simulink model "CDMA_AWGN"  (Simulink 7.6)
settings: Solver=ode45  StartTime=0.0  StopTime=inf  RelTol=1e-3
libraries: commdigbbndpm3 x11, commseqgen2 x8, dspsigops x6, commfilt2 x6, commchan3 x2, commrandsrc2 x2, commsink2 x1
settings Model: Creator=Administrator  LastModifiedBy=Administrator

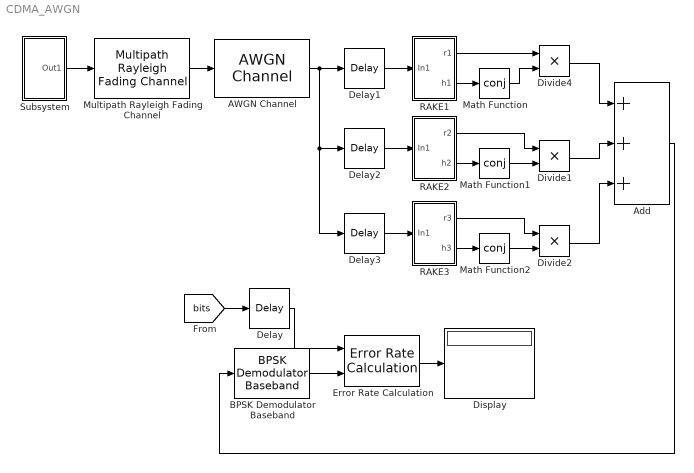
== system CDMA_AWGN ==
  AWGN Channel : commchan3/AWGN Channel  SystemSampleTime=-1  InputProcessing=Columns as channels (frame based)  seed=67  noiseMode="Signal to noise ratio  (Eb/No)"  EbNodB=4  EsNodB=10  SNRdB=10  bitsPerSym=1  Ps=1  Tsym=1e-6  variance=1
  Add : Sum  Inputs=+++
  BPSK Demodulator Baseband : commdigbbndpm3/BPSK Demodulator Baseband  DialogController=commDDGCreate  DialogControllerArgs=DataTag1  Ph=0  DecType=Hard decision  VarSource=Dialog  Variance=1  outDtype=Inherit via internal rule  derotateFactorWordLen=16
  Delay : dspsigops/Delay  InputProcessing=Columns as channels (frame based)  dly_unit=Samples  delay=1  ic_detail=off  dif_ic_for_ch=off  dif_ic_for_dly=off  ic=0  reset_popup=None
  Delay1 : dspsigops/Delay  InputProcessing=Columns as channels (frame based)  dly_unit=Samples  delay=63  ic_detail=off  dif_ic_for_ch=off  dif_ic_for_dly=off  ic=0  reset_popup=None
  Delay2 : dspsigops/Delay  InputProcessing=Columns as channels (frame based)  dly_unit=Samples  delay=62  ic_detail=off  dif_ic_for_ch=off  dif_ic_for_dly=off  ic=0  reset_popup=None
  Delay3 : dspsigops/Delay  InputProcessing=Columns as channels (frame based)  dly_unit=Samples  delay=61  ic_detail=off  dif_ic_for_ch=off  dif_ic_for_dly=off  ic=0  reset_popup=None
  Display : Display
  Divide1 : Product  Inputs=**
  Divide2 : Product  Inputs=**
  Divide4 : Product  Inputs=**
  Error Rate Calculation : commsink2/Error Rate Calculation  N=0  st_delay=10  cp_mode=Entire frame  subframe=[]  PMode=Port  WsName=ErrorVec  RsMode2=off  stop=off  numErr=100  maxBits=1e6
  Math Function : Math  Operator=conj  SaturateOnIntegerOverflow=on
  Math Function1 : Math  Operator=conj  SaturateOnIntegerOverflow=on
  Math Function2 : Math  Operator=conj  SaturateOnIntegerOverflow=on
  Multipath Rayleigh Fading Channel : commchan3/Multipath Rayleigh Fading Channel  SystemSampleTime=-1  maxDopplerShift=40  spectrumType=Jakes  sigmaGaussian=1/sqrt(2)  coeffRounded=[1 -1.72 0.785]  freqMinMaxRJakes=[0 1]  freqMinMaxAJakes=[0 1]  sigmaGaussian1=1/sqrt(2)  sigmaGaussian2=1/sqrt(2)  centerFreqGaussian1=0.0  centerFreqGaussian2=0.0  gainGaussian1=0.5  gainGaussian2=0.5  coeffBell=9  dopplerSpectrum=doppler.jakes  pathDelays=[0 1e-6/63 2e-6/63]  avgPathGaindB=[0 -3 -6]  normalizePathGains=on  seed=73  enableProbe=0  openVisAtStart=off  outPathGains=off  outDelay=off
  RAKE1 : Subsystem
  RAKE2 : Subsystem
  RAKE3 : Subsystem
  Subsystem : Subsystem
  wires:
  BPSK Demodulator Baseband/1 -> Error Rate Calculation/2
  Error Rate Calculation/1 -> Display/1
  Subsystem/1(Out1) -> Multipath Rayleigh Fading Channel/1
  Multipath Rayleigh Fading Channel/1 -> AWGN Channel/1
  AWGN Channel/1 -> Delay2/1, Delay3/1, Delay1/1
  Divide4/1 -> Add/1
  Divide1/1 -> Add/2
  Divide2/1 -> Add/3
  Delay1/1 -> RAKE1/1(In1)
  Delay2/1 -> RAKE2/1(In1)
  Delay3/1 -> RAKE3/1(In1)
  RAKE1/1(r1) -> Divide4/1
  RAKE1/2(h1) -> Math Function/1
  Math Function/1 -> Divide4/2
  RAKE2/1(r2) -> Divide1/1
  RAKE2/2(h2) -> Math Function1/1
  Math Function1/1 -> Divide1/2
  RAKE3/1(r3) -> Divide2/1
  RAKE3/2(h3) -> Math Function2/1
  Math Function2/1 -> Divide2/2
  [bits] -> Delay/1
  Add/1 -> BPSK Demodulator Baseband/1
  Delay/1 -> Error Rate Calculation/1

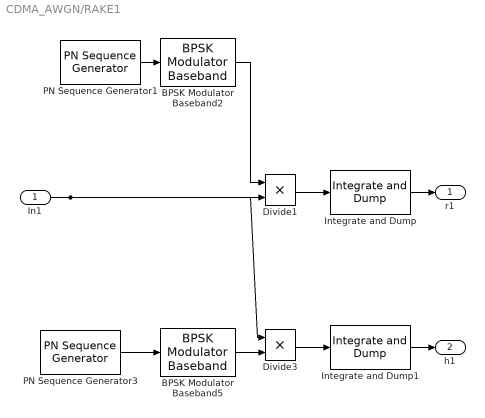
== system CDMA_AWGN/RAKE1 ==
  In1 : Inport
  BPSK Modulator Baseband2 : commdigbbndpm3/BPSK Modulator Baseband  DialogController=commDDGCreate  DialogControllerArgs=DataTag6  SystemSampleTime=-1  Ph=0  outDtype=double  outWordLen=16  outUDDataType=sfix(16)  outFracLenMode=Best precision  outFracLen=15
  BPSK Modulator Baseband5 : commdigbbndpm3/BPSK Modulator Baseband  DialogController=commDDGCreate  DialogControllerArgs=DataTag7  SystemSampleTime=-1  Ph=0  outDtype=double  outWordLen=16  outUDDataType=sfix(16)  outFracLenMode=Best precision  outFracLen=15
  Divide1 : Product  Inputs=**
  Divide3 : Product  Inputs=**
  Integrate and Dump : commfilt2/Integrate and Dump  DialogController=commDDGCreate  DialogControllerArgs=DataTag8  obssamples=63  offsetsamples=0  nodump=off  roundingMode=Floor  overflowMode=off
  Integrate and Dump1 : commfilt2/Integrate and Dump  DialogController=commDDGCreate  DialogControllerArgs=DataTag9  obssamples=63  offsetsamples=0  nodump=off  roundingMode=Floor  overflowMode=off
  PN Sequence Generator1 : commseqgen2/PN Sequence Generator  poly=[1 0 0 0 0 1 1]  ini_sta=[0 0 0 0 0 1]  outBitMaskSource=Dialog parameter  shift=0  Ts=1e-6/63  frameBased=on  sampPerFrame=63  reset=off  bitPackedOutputs=off  outDataType=double  numPackedBits=8  bitPackDataSigned=off  bitPackedOutDType=double
  PN Sequence Generator3 : commseqgen2/PN Sequence Generator  poly=[1 0 0 0 0 1 1]  ini_sta=[0 1 0 1 0 1]  outBitMaskSource=Dialog parameter  shift=0  Ts=1e-6/63  frameBased=on  sampPerFrame=63  reset=off  bitPackedOutputs=off  outDataType=double  numPackedBits=8  bitPackDataSigned=off  bitPackedOutDType=double
  r1 : Outport
  h1 : Outport  Port=2
  wires:
  PN Sequence Generator1/1 -> BPSK Modulator Baseband2/1
  Divide1/1 -> Integrate and Dump/1
  BPSK Modulator Baseband2/1 -> Divide1/1
  In1/1 -> Divide3/1, Divide1/2
  PN Sequence Generator3/1 -> BPSK Modulator Baseband5/1
  BPSK Modulator Baseband5/1 -> Divide3/2
  Divide3/1 -> Integrate and Dump1/1
  Integrate and Dump/1 -> r1/1
  Integrate and Dump1/1 -> h1/1

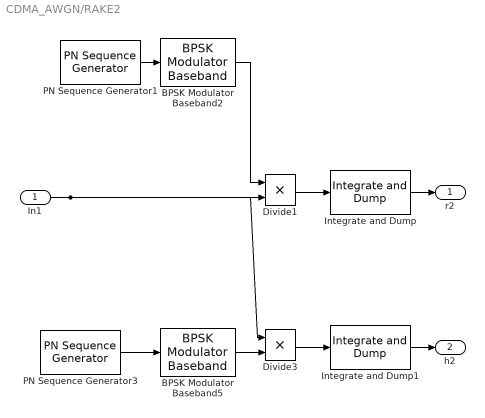
== system CDMA_AWGN/RAKE2 ==
  In1 : Inport
  BPSK Modulator Baseband2 : commdigbbndpm3/BPSK Modulator Baseband  DialogController=commDDGCreate  DialogControllerArgs=DataTag10  SystemSampleTime=-1  Ph=0  outDtype=double  outWordLen=16  outUDDataType=sfix(16)  outFracLenMode=Best precision  outFracLen=15
  BPSK Modulator Baseband5 : commdigbbndpm3/BPSK Modulator Baseband  DialogController=commDDGCreate  DialogControllerArgs=DataTag11  SystemSampleTime=-1  Ph=0  outDtype=double  outWordLen=16  outUDDataType=sfix(16)  outFracLenMode=Best precision  outFracLen=15
  Divide1 : Product  Inputs=**
  Divide3 : Product  Inputs=**
  Integrate and Dump : commfilt2/Integrate and Dump  DialogController=commDDGCreate  DialogControllerArgs=DataTag12  obssamples=63  offsetsamples=0  nodump=off  roundingMode=Floor  overflowMode=off
  Integrate and Dump1 : commfilt2/Integrate and Dump  DialogController=commDDGCreate  DialogControllerArgs=DataTag13  obssamples=63  offsetsamples=0  nodump=off  roundingMode=Floor  overflowMode=off
  PN Sequence Generator1 : commseqgen2/PN Sequence Generator  poly=[1 0 0 0 0 1 1]  ini_sta=[0 0 0 0 0 1]  outBitMaskSource=Dialog parameter  shift=0  Ts=1e-6/63  frameBased=on  sampPerFrame=63  reset=off  bitPackedOutputs=off  outDataType=double  numPackedBits=8  bitPackDataSigned=off  bitPackedOutDType=double
  PN Sequence Generator3 : commseqgen2/PN Sequence Generator  poly=[1 0 0 0 0 1 1]  ini_sta=[0 1 0 1 0 1]  outBitMaskSource=Dialog parameter  shift=0  Ts=1e-6/63  frameBased=on  sampPerFrame=63  reset=off  bitPackedOutputs=off  outDataType=double  numPackedBits=8  bitPackDataSigned=off  bitPackedOutDType=double
  r2 : Outport
  h2 : Outport  Port=2
  wires:
  Integrate and Dump1/1 -> h2/1
  Integrate and Dump/1 -> r2/1
  Divide3/1 -> Integrate and Dump1/1
  BPSK Modulator Baseband5/1 -> Divide3/2
  PN Sequence Generator3/1 -> BPSK Modulator Baseband5/1
  In1/1 -> Divide1/2, Divide3/1
  BPSK Modulator Baseband2/1 -> Divide1/1
  Divide1/1 -> Integrate and Dump/1
  PN Sequence Generator1/1 -> BPSK Modulator Baseband2/1

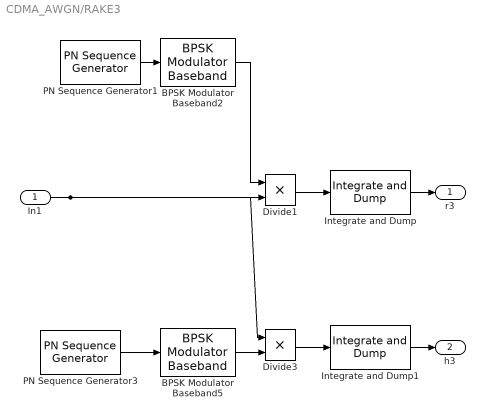
== system CDMA_AWGN/RAKE3 ==
  In1 : Inport
  BPSK Modulator Baseband2 : commdigbbndpm3/BPSK Modulator Baseband  DialogController=commDDGCreate  DialogControllerArgs=DataTag14  SystemSampleTime=-1  Ph=0  outDtype=double  outWordLen=16  outUDDataType=sfix(16)  outFracLenMode=Best precision  outFracLen=15
  BPSK Modulator Baseband5 : commdigbbndpm3/BPSK Modulator Baseband  DialogController=commDDGCreate  DialogControllerArgs=DataTag15  SystemSampleTime=-1  Ph=0  outDtype=double  outWordLen=16  outUDDataType=sfix(16)  outFracLenMode=Best precision  outFracLen=15
  Divide1 : Product  Inputs=**
  Divide3 : Product  Inputs=**
  Integrate and Dump : commfilt2/Integrate and Dump  DialogController=commDDGCreate  DialogControllerArgs=DataTag16  obssamples=63  offsetsamples=0  nodump=off  roundingMode=Floor  overflowMode=off
  Integrate and Dump1 : commfilt2/Integrate and Dump  DialogController=commDDGCreate  DialogControllerArgs=DataTag17  obssamples=63  offsetsamples=0  nodump=off  roundingMode=Floor  overflowMode=off
  PN Sequence Generator1 : commseqgen2/PN Sequence Generator  poly=[1 0 0 0 0 1 1]  ini_sta=[0 0 0 0 0 1]  outBitMaskSource=Dialog parameter  shift=0  Ts=1e-6/63  frameBased=on  sampPerFrame=63  reset=off  bitPackedOutputs=off  outDataType=double  numPackedBits=8  bitPackDataSigned=off  bitPackedOutDType=double
  PN Sequence Generator3 : commseqgen2/PN Sequence Generator  poly=[1 0 0 0 0 1 1]  ini_sta=[0 1 0 1 0 1]  outBitMaskSource=Dialog parameter  shift=0  Ts=1e-6/63  frameBased=on  sampPerFrame=63  reset=off  bitPackedOutputs=off  outDataType=double  numPackedBits=8  bitPackDataSigned=off  bitPackedOutDType=double
  r3 : Outport
  h3 : Outport  Port=2
  wires:
  PN Sequence Generator1/1 -> BPSK Modulator Baseband2/1
  Divide1/1 -> Integrate and Dump/1
  BPSK Modulator Baseband2/1 -> Divide1/1
  In1/1 -> Divide3/1, Divide1/2
  PN Sequence Generator3/1 -> BPSK Modulator Baseband5/1
  BPSK Modulator Baseband5/1 -> Divide3/2
  Divide3/1 -> Integrate and Dump1/1
  Integrate and Dump/1 -> r3/1
  Integrate and Dump1/1 -> h3/1

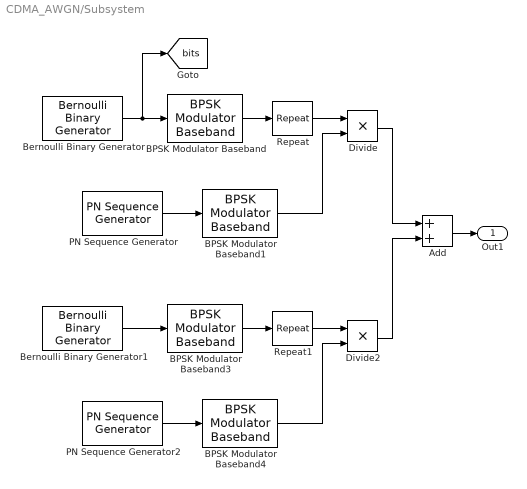
== system CDMA_AWGN/Subsystem ==
  Add : Sum
  BPSK Modulator Baseband : commdigbbndpm3/BPSK Modulator Baseband  DialogController=commDDGCreate  DialogControllerArgs=DataTag18  SystemSampleTime=-1  Ph=0  outDtype=double  outWordLen=16  outUDDataType=sfix(16)  outFracLenMode=Best precision  outFracLen=15
  BPSK Modulator Baseband1 : commdigbbndpm3/BPSK Modulator Baseband  DialogController=commDDGCreate  DialogControllerArgs=DataTag19  SystemSampleTime=-1  Ph=0  outDtype=double  outWordLen=16  outUDDataType=sfix(16)  outFracLenMode=Best precision  outFracLen=15
  BPSK Modulator Baseband3 : commdigbbndpm3/BPSK Modulator Baseband  DialogController=commDDGCreate  DialogControllerArgs=DataTag20  SystemSampleTime=-1  Ph=0  outDtype=double  outWordLen=16  outUDDataType=sfix(16)  outFracLenMode=Best precision  outFracLen=15
  BPSK Modulator Baseband4 : commdigbbndpm3/BPSK Modulator Baseband  DialogController=commDDGCreate  DialogControllerArgs=DataTag21  SystemSampleTime=-1  Ph=0  outDtype=double  outWordLen=16  outUDDataType=sfix(16)  outFracLenMode=Best precision  outFracLen=15
  Bernoulli Binary Generator : commrandsrc2/Bernoulli Binary Generator  DialogController=commDDGCreate  DialogControllerArgs=DataTag22  SystemSampleTime=-1  P=0.5  seed=61  Ts=1e-6  frameBased=off  sampPerFrame=1  orient=off  outDataType=double
  Bernoulli Binary Generator1 : commrandsrc2/Bernoulli Binary Generator  DialogController=commDDGCreate  DialogControllerArgs=DataTag23  SystemSampleTime=-1  P=1  seed=61  Ts=1e-6  frameBased=off  sampPerFrame=1  orient=off  outDataType=double
  Divide : Product  Inputs=**
  Divide2 : Product  Inputs=**
  PN Sequence Generator : commseqgen2/PN Sequence Generator  poly=[1 0 0 0 0 1 1]  ini_sta=[0 0 0 0 0 1]  outBitMaskSource=Dialog parameter  shift=0  Ts=1e-6/63  frameBased=on  sampPerFrame=63  reset=off  bitPackedOutputs=off  outDataType=double  numPackedBits=8  bitPackDataSigned=off  bitPackedOutDType=double
  PN Sequence Generator2 : commseqgen2/PN Sequence Generator  poly=[1 0 0 0 0 1 1]  ini_sta=[0 1 0 1 0 1]  outBitMaskSource=Dialog parameter  shift=0  Ts=1e-6/63  frameBased=on  sampPerFrame=63  reset=off  bitPackedOutputs=off  outDataType=double  numPackedBits=8  bitPackDataSigned=off  bitPackedOutDType=double
  Repeat : dspsigops/Repeat  N=63  InputProcessing=Columns as channels (frame based)  RateOptions=Enforce single-rate processing  ic=0  mode=Unused parameter value
  Repeat1 : dspsigops/Repeat  N=63  InputProcessing=Columns as channels (frame based)  RateOptions=Enforce single-rate processing  ic=0  mode=Unused parameter value
  Out1 : Outport
  tag scope: bits=global
  wires:
  Bernoulli Binary Generator/1 -> BPSK Modulator Baseband/1, [bits]
  BPSK Modulator Baseband/1 -> Repeat/1
  Repeat/1 -> Divide/1
  PN Sequence Generator/1 -> BPSK Modulator Baseband1/1
  BPSK Modulator Baseband1/1 -> Divide/2
  Bernoulli Binary Generator1/1 -> BPSK Modulator Baseband3/1
  BPSK Modulator Baseband3/1 -> Repeat1/1
  Repeat1/1 -> Divide2/1
  PN Sequence Generator2/1 -> BPSK Modulator Baseband4/1
  BPSK Modulator Baseband4/1 -> Divide2/2
  Divide/1 -> Add/1
  Divide2/1 -> Add/2
  Add/1 -> Out1/1
